simulink model "Project_LQR_MODEL_HIL"  (R2023b)
settings: Solver=ode3  StartTime=0.0  StopTime=inf  FixedStep=0.001  RelTol=1e-3  EnableMultiTasking=on
StartFcn:
  | theta_o='LQR_MODEL/Out_1';
  | theta_o_dot='LQR_MODEL/Out_2';
  | theta_1='LQR_MODEL/Out_3';
  | theta_1_dot='LQR_MODEL/Out_4';
  | ctrl_action='LQR_MODEL/Out_5';
  | event='PostOutputs';
  | listener=@update_app_designer;
  | h1=add_exec_event_listener(theta_o,event,listener);
  | h2=add_exec_event_listener(theta_o_dot,event,listener);
  | h3=add_exec_event_listener(theta_1,event,listener);
  | h4=add_exec_event_listener(theta_1_dot,event,listener);
  | h5=add_exec_event_listener(ctrl_action,event,listener);
undefined symbols (not defined in the file or in its folder): k, k1, k2, k3, k4
libraries: simulink_extras x4, arduinolib x3, eeGeneralControl x2
settings Model: FPTRunName=Active  SimulationMode=external  ExtModeTrigDuration=2  Creator=AHMED MOHSEN  LastModifiedBy=AHMED MOHSEN
settings SolverCC: AlgebraicLoopSolver=TrustRegion
settings DataIOCC: LimitDataPoints=on  SaveFormat=Array
settings OptimizationCC: ReuseModelBlockBuffer=off  ExpressionDepthLimit=2147483647  LifeSpan=Inf  MaxStackSize=64
settings DebuggingCC: UnderspecifiedInitializationDetection=Classic  MergeDetectMultiDrivingBlocksExec=none  FcnCallInpInsideContextMsg=warning  UnconnectedInputMsg=warning  UnconnectedOutputMsg=warning  UnconnectedLineMsg=warning  AllowSymbolicDim=off  StateNameClashWarn=warning  SFUnexpectedBacktrackingDiag=warning  SFNoUnconditionalDefaultTransitionDiag=warning  SFExecutionAtInitializationDiag=none  ArithmeticOperatorsInVariantConditions=warning
settings HardwareCC: ProdBitPerInt=16  ProdBitPerPointer=16  ProdBitPerSizeT=16  ProdBitPerPtrDiffT=16  ProdLargestAtomicFloat=None  ProdWordSize=8  ProdHWDeviceType=Atmel->AVR  UseEmbeddedCoderFeatures=off  UseSimulinkCoderFeatures=off
settings ModelReferenceCC: EnableRefExpFcnMdlSchedulingChecks=on  PropagateSignalLabelsOutOfModel=off
settings SFSimCC: SimUseLocalCustomCode=off  CustomCodeUndefinedFunction=UseInterfaceOnly
settings RTWCC: Description=Embedded Coder  SystemTargetFile=ert.tlc  HardwareBoard=Arduino Mega 2560  TemplateMakefile=ert_default_tmf  GenerateReport=on  RTWVerbose=off  RTWUseLocalCustomCode=off  Toolchain=Arduino AVR  BuildConfiguration=Faster Runs  LaunchReport=on
settings CodeAppCC: ForceParamTrailComments=on  OperatorAnnotations=on  StateflowObjectComments=on  MATLABSourceComments=on
settings ERTTargetCC: MultiwordLength=2048  ERTCustomFileBanners=off  SupportContinuousTime=on  SupportNonInlinedSFcns=on  RemoveResetFunc=off  ModelStepFunctionPrototypeControlCompliant=off
settings ConfigComp: CovMetricSettings=dw  CovSaveCumulativeToWorkspaceVar=on  CovSaveSingleToWorkspaceVar=on  CovExternalEMLEnable=off  CovSFcnEnable=off

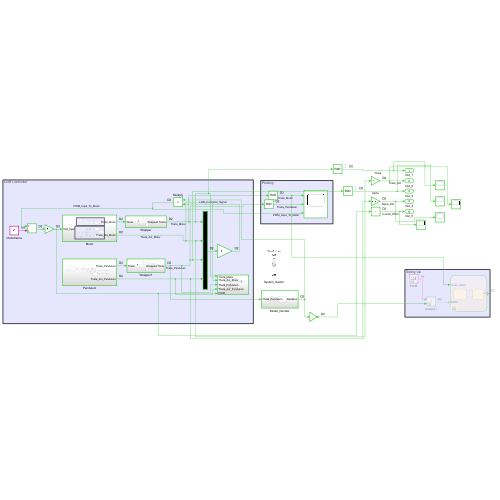
[thumbnail: Simulink's stored preview of the top-level diagram]
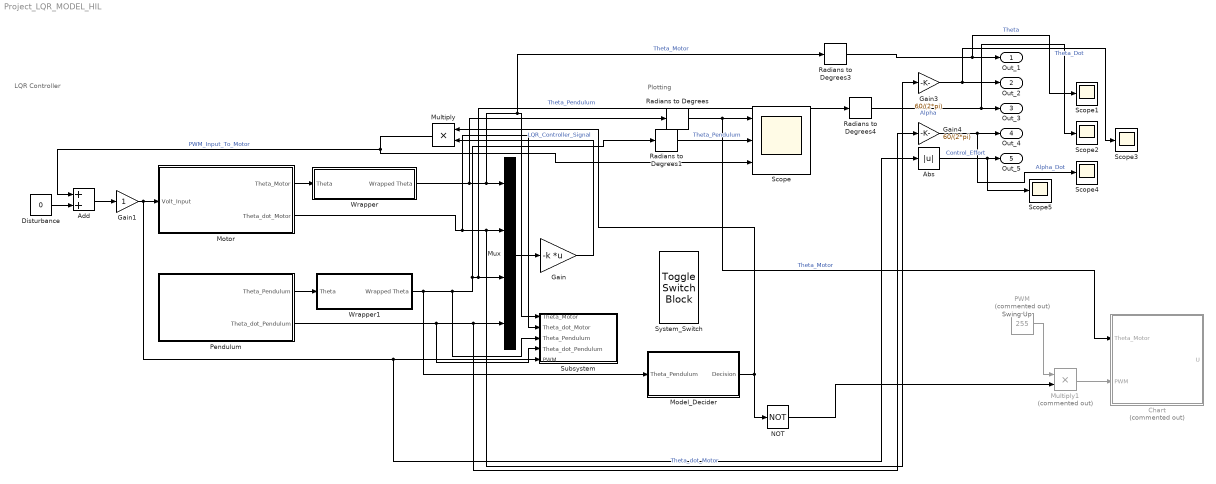
== system Project_LQR_MODEL_HIL ==
  note: Plotting
  note: Swing Up
  note: LQR Controller
  Abs : Abs  SaturateOnIntegerOverflow=off
  Add : Sum
  Chart : Stateflow chart  Commented=on  TreatAsAtomicUnit=on
  Disturbance : Constant  Value=0
  Gain : Gain  Gain=-k  Multiplication=Matrix(K*u)
  Gain1 : Gain
  Gain3 : Gain  Gain=60/(2*pi)
  Gain4 : Gain  Gain=60/(2*pi)
  Model_Decider : Subsystem
  Motor : Subsystem
  Multiply : Product  Inputs=**
  Multiply1 : Product  Commented=on  Inputs=**
  Mux : Mux
  NOT : Logic  Operator=NOT  IconShape=distinctive  AllPortsSameDT=off  OutDataTypeStr=boolean
  PWM : Constant  Commented=on  Value=255
  Pendulum : Subsystem
  Radians to Degrees{,1,3..4} (4 alike) : simulink_extras/Transformations/Radians to Degrees
  Scope : Scope  NumInputPorts=3
  Scope{1..5} (5 alike) : Scope
  Subsystem : Subsystem
  System_Switch : ToggleSwitchBlock
      settings: Values={{'Off', 'On'}, [0 1]}
  Wrapper : Subsystem
  Wrapper1 : Subsystem
  Out_1 : Outport
  Out_2 : Outport  Port=2
  Out_3 : Outport  Port=3
  Out_4 : Outport  Port=4
  Out_5 : Outport  Port=5
  wires:
  Mux/1 -> Gain/1
  Multiply/1 -> Add/1, Scope/3  "PWM_Input_To_Motor"
  Pendulum/2(Theta_dot_Pendulum) -> Subsystem/4(Theta_dot_Pendulum), Gain4/1, Mux/4
  Pendulum/1(Theta_Pendulum) -> Wrapper1/1(Theta)
  Motor/1(Theta_Motor) -> Wrapper/1(Theta)
  Gain/1 -> Multiply/2  "LQR_Controller_Signal"
  Motor/2(Theta_dot_Motor) -> Subsystem/2(Theta_dot_Motor), Gain3/1, Mux/2  "Theta_dot_Motor"
  Wrapper/1(Wrapped Theta) -> Radians to Degrees/1, Radians to Degrees3/1, Subsystem/1(Theta_Motor), Mux/1  "Theta_Motor"
  Wrapper1/1(Wrapped Theta) -> Model_Decider/1(Theta_Pendulum), Subsystem/3(Theta_Pendulum), Radians to Degrees4/1, Mux/3, Radians to Degrees1/1  "Theta_Pendulum"
  Radians to Degrees/1 -> Chart/1(Theta_Motor), Scope/1  "Theta_Motor"
  Radians to Degrees1/1 -> Scope/2  "Theta_Pendulum"
  NOT/1 -> Multiply1/2
  PWM/1 -> Multiply1/1
  Multiply1/1 -> Chart/2(PWM)
  Add/1 -> Gain1/1
  Model_Decider/1(Decision) -> NOT/1, Multiply/1
  Radians to Degrees3/1 -> Scope1/1, Out_1/1  "Theta"
  Gain3/1 -> Scope3/1, Out_2/1  "Theta_Dot"
  Radians to Degrees4/1 -> Scope2/1, Out_3/1  "Alpha"
  Gain1/1 -> Abs/1, Subsystem/5(PWM), Motor/1(Volt_Input)
  Abs/1 -> Scope5/1, Out_5/1  "Control_Effort"
  Gain4/1 -> Scope4/1, Out_4/1  "Alpha_Dot"
  Disturbance/1 -> Add/2

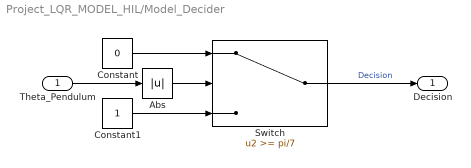
== system Project_LQR_MODEL_HIL/Model_Decider ==
  Theta_Pendulum : Inport
  Abs : Abs  SaturateOnIntegerOverflow=off
  Constant : Constant  Value=0
  Constant1 : Constant
  Switch : Switch  Threshold=pi/7  SaturateOnIntegerOverflow=off  InputSameDT=off
  Decision : Outport
  wires:
  Constant/1 -> Switch/1
  Abs/1 -> Switch/2
  Constant1/1 -> Switch/3
  Switch/1 -> Decision/1  "Decision"
  Theta_Pendulum/1 -> Abs/1

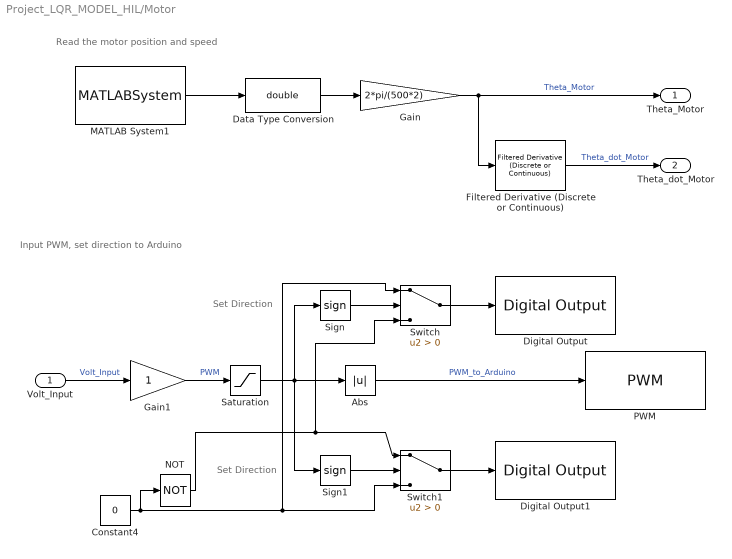
== system Project_LQR_MODEL_HIL/Motor ==
  note: Set Direction
  note: Input PWM, set direction to Arduino
  note: Read the motor position and speed
  note: Set Direction
  Volt_Input : Inport
  Abs : Abs  SaturateOnIntegerOverflow=off
  Constant4 : Constant  Value=0
  Data Type Conversion : DataTypeConversion  OutDataTypeStr=double  SaturateOnIntegerOverflow=off  RndMeth=Floor
  Digital Output : arduinolib/Digital Output  pinNumber=9  Direction=output  blockPlatform=arduino
  Digital Output1 : arduinolib/Digital Output  pinNumber=10  Direction=output  blockPlatform=arduino
  Filtered Derivative (Discrete or Continuous) : eeGeneralControl/Filtered Derivative (Discrete or Continuous)  K=1  T=0.001  B=inf  A=-inf  minRatio=10  init_option=Inherited from block input  x0=0  Ts=-1
      settings: LibrarySourceBlock=|
      | ee_sl_lib/General Control/Filtered Derivative
      | (Discrete or Continuous)
  Gain : Gain  Gain=2*pi/(500*2)
  Gain1 : Gain
  MATLAB System1 : MATLABSystem  System=Encoder_arduino  Encoder=1  PinA=2  PinB=4  SampleTime=0.01
      mask Type: Encoder_arduino
      mask Display:
      | disp('Encoder');
      | port_label('output',1,'y');
  NOT : Logic  Operator=NOT  IconShape=distinctive  AllPortsSameDT=off  OutDataTypeStr=boolean
  PWM : arduinolib/PWM  pinNumber=8  frequencyType=Default  desiredFrequency=490.2  achievableFrequency=490.2
  Saturation : Saturate  UpperLimit=255  LowerLimit=-255
  Sign : Signum
  Sign1 : Signum
  Switch : Switch  Criteria=u2 > Threshold  SaturateOnIntegerOverflow=off  InputSameDT=off
  Switch1 : Switch  Criteria=u2 > Threshold  SaturateOnIntegerOverflow=off  InputSameDT=off
  Theta_Motor : Outport
  Theta_dot_Motor : Outport  Port=2
  wires:
  MATLAB System1/1 -> Data Type Conversion/1
  Data Type Conversion/1 -> Gain/1
  Gain/1 -> Filtered Derivative (Discrete or Continuous)/1, Theta_Motor/1  "Theta_Motor"
  Filtered Derivative (Discrete or Continuous)/1 -> Theta_dot_Motor/1  "Theta_dot_Motor"
  Volt_Input/1 -> Gain1/1  "Volt_Input"
  Sign/1 -> Switch/2
  Constant4/1 -> Switch/1, Switch1/3, NOT/1
  Sign1/1 -> Switch1/2
  Saturation/1 -> Abs/1, Sign1/1, Sign/1
  NOT/1 -> Switch/3, Switch1/1
  Abs/1 -> PWM/1  "PWM_to_Arduino"
  Switch/1 -> Digital Output/1
  Switch1/1 -> Digital Output1/1
  Gain1/1 -> Saturation/1  "PWM"

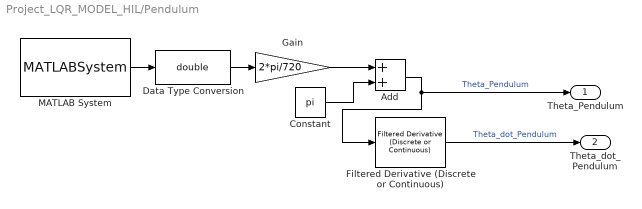
== system Project_LQR_MODEL_HIL/Pendulum ==
  Add : Sum
  Constant : Constant  Value=pi
  Data Type Conversion : DataTypeConversion  OutDataTypeStr=double  SaturateOnIntegerOverflow=off  RndMeth=Floor
  Filtered Derivative (Discrete or Continuous) : eeGeneralControl/Filtered Derivative (Discrete or Continuous)  K=1  T=0.001  B=inf  A=-inf  minRatio=10  init_option=Inherited from block input  x0=0  Ts=-1
      settings: LibrarySourceBlock=|
      | ee_sl_lib/General Control/Filtered Derivative
      | (Discrete or Continuous)
  Gain : Gain  Gain=2*pi/720
  MATLAB System : MATLABSystem  System=Encoder_arduino  Encoder=0  PinA=3  PinB=5  SampleTime=0.01
      mask Type: Encoder_arduino
      mask Display:
      | disp('Encoder');
      | port_label('output',1,'y');
  Theta_Pendulum : Outport
  Theta_dot_Pendulum : Outport  Port=2
  wires:
  MATLAB System/1 -> Data Type Conversion/1
  Data Type Conversion/1 -> Gain/1
  Gain/1 -> Add/1
  Constant/1 -> Add/2
  Add/1 -> Theta_Pendulum/1, Filtered Derivative (Discrete or Continuous)/1  "Theta_Pendulum"
  Filtered Derivative (Discrete or Continuous)/1 -> Theta_dot_Pendulum/1  "Theta_dot_Pendulum"

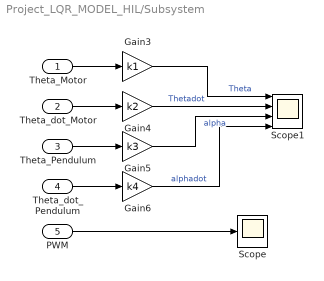
== system Project_LQR_MODEL_HIL/Subsystem ==
  Theta_Motor : Inport
  Theta_dot_Motor : Inport  Port=2
  Theta_Pendulum : Inport  Port=3
  Theta_dot_Pendulum : Inport  Port=4
  PWM : Inport  Port=5
  Gain3 : Gain  Gain=k1
  Gain4 : Gain  Gain=k2
  Gain5 : Gain  Gain=k3
  Gain6 : Gain  Gain=k4
  Scope : Scope
  Scope1 : Scope  NumInputPorts=4
  wires:
  Gain3/1 -> Scope1/1  "Theta"
  Gain5/1 -> Scope1/3  "alpha"
  Gain4/1 -> Scope1/2  "Thetadot"
  Gain6/1 -> Scope1/4  "alphadot"
  Theta_dot_Motor/1 -> Gain4/1
  Theta_Motor/1 -> Gain3/1
  Theta_dot_Pendulum/1 -> Gain6/1
  Theta_Pendulum/1 -> Gain5/1
  PWM/1 -> Scope/1

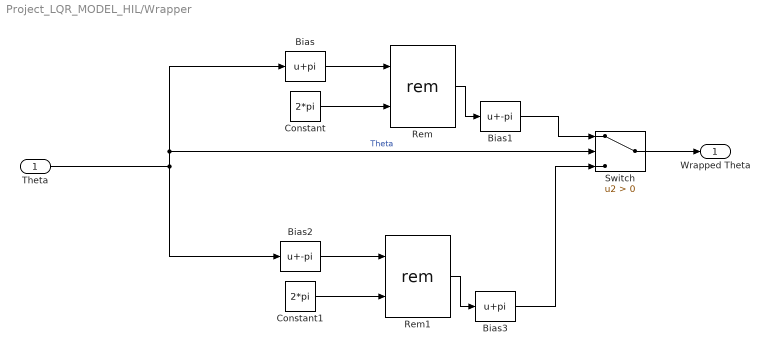
== system Project_LQR_MODEL_HIL/Wrapper ==
  Theta : Inport
  Bias : Bias  Bias=pi  SaturateOnIntegerOverflow=off
  Bias1 : Bias  Bias=-pi  SaturateOnIntegerOverflow=off
  Bias2 : Bias  Bias=-pi  SaturateOnIntegerOverflow=off
  Bias3 : Bias  Bias=pi  SaturateOnIntegerOverflow=off
  Constant : Constant  Value=2*pi
  Constant1 : Constant  Value=2*pi
  Rem : Math  Operator=rem
  Rem1 : Math  Operator=rem
  Switch : Switch  Criteria=u2 > Threshold  SaturateOnIntegerOverflow=off  InputSameDT=off
  Wrapped Theta : Outport
  wires:
  Theta/1 -> Bias2/1, Bias/1, Switch/2  "Theta"
  Bias/1 -> Rem/1
  Constant/1 -> Rem/2
  Rem/1 -> Bias1/1
  Bias1/1 -> Switch/1
  Constant1/1 -> Rem1/2
  Rem1/1 -> Bias3/1
  Bias2/1 -> Rem1/1
  Bias3/1 -> Switch/3
  Switch/1 -> Wrapped Theta/1

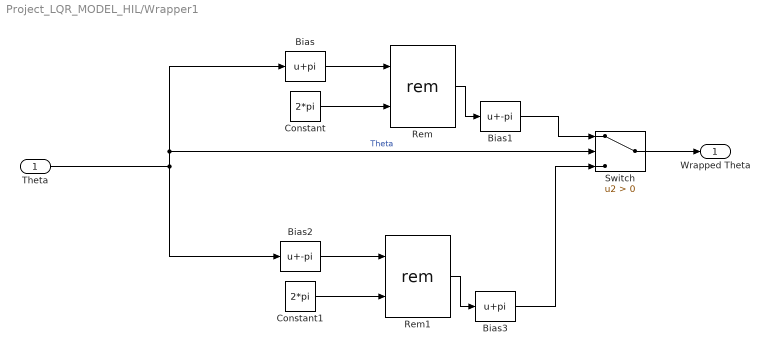
== system Project_LQR_MODEL_HIL/Wrapper1 ==
  Theta : Inport
  Bias : Bias  Bias=pi  SaturateOnIntegerOverflow=off
  Bias1 : Bias  Bias=-pi  SaturateOnIntegerOverflow=off
  Bias2 : Bias  Bias=-pi  SaturateOnIntegerOverflow=off
  Bias3 : Bias  Bias=pi  SaturateOnIntegerOverflow=off
  Constant : Constant  Value=2*pi
  Constant1 : Constant  Value=2*pi
  Rem : Math  Operator=rem
  Rem1 : Math  Operator=rem
  Switch : Switch  Criteria=u2 > Threshold  SaturateOnIntegerOverflow=off  InputSameDT=off
  Wrapped Theta : Outport
  wires:
  Theta/1 -> Bias2/1, Bias/1, Switch/2  "Theta"
  Bias/1 -> Rem/1
  Constant/1 -> Rem/2
  Rem/1 -> Bias1/1
  Bias1/1 -> Switch/1
  Constant1/1 -> Rem1/2
  Rem1/1 -> Bias3/1
  Bias2/1 -> Rem1/1
  Bias3/1 -> Switch/3
  Switch/1 -> Wrapped Theta/1

== stateflow chart Project_LQR_MODEL_HIL/Chart ==
  state CW
    entry:
    U=-PWM
  state CCW
    entry:
    U=PWM
  (default) -> CW
  CW -> CCW : [Theta_Motor>=30]
  CCW -> CW : [Theta_Motor<=0]
  data: Theta_Motor input; PWM input; U output
